simulink model "sum_oddmdl"  (R2021a)
settings: Solver=VariableStepAuto  StartTime=0.0  StopTime=10.0  RelTol=1e-3
settings Model: Creator=Acer  LastModifiedBy=Acer

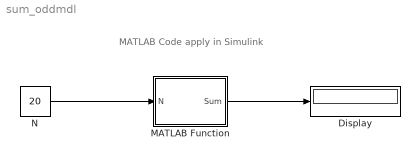
== system sum_oddmdl ==
  note: MATLAB Code apply in Simulink
  Display : Display
  MATLAB Function : MATLAB Function  TreatAsAtomicUnit=on
  N : Constant  Value=20
  wires:
  N/1 -> MATLAB Function/1(N)
  MATLAB Function/1(Sum) -> Display/1

== matlab function sum_oddmdl/MATLAB Function ==
  data: N input; Sum output
function Sum = fcn(N)
Sum=0; count=1;
while ne(count,N)
    if mod(count,2)~=0
        Sum=Sum+count;
    end
    count=count+1;
end
end
